simulink library "headingSetpointNumerical_cl"  (R2018b)
settings: Solver=VariableStepAuto  StartTime=0.0  StopTime=10.0  RelTol=1e-3
undefined symbols (not defined in the file): initialPathPosition_none
libraries: flatlandHeading_ul x1, offsetLeadDistance_ul x1, pathPositionNumerical_ul x1, pathProjectionNumerical_ul x1
settings Model: Creator=mcobb  LastModifiedBy=mitch
settings DebuggingCC: LibraryContextMissingDiagnostic=none
settings SFSimCC: SimUseLocalCustomCode=off
settings RTWCC: RTWUseLocalCustomCode=off

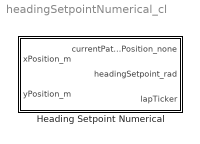
== system headingSetpointNumerical_cl ==
  Heading Setpoint Numerical : Subsystem

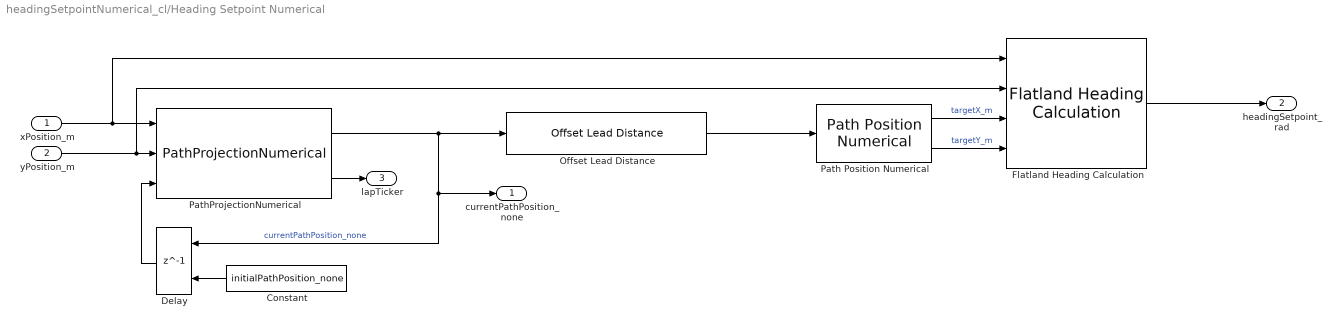
== system headingSetpointNumerical_cl/Heading Setpoint Numerical ==
  xPosition_m : Inport
  yPosition_m : Inport  Port=2
  Constant : Constant  Value=initialPathPosition_none
  Delay : Delay  DelayLength=1  InitialConditionSource=Input port  InitialCondition=0
      settings: InputPortMap=u0,p4
  Flatland Heading Calculation : flatlandHeading_ul/Flatland Heading Calculation  SystemSampleTime=-1
  Offset Lead Distance : offsetLeadDistance_ul/Offset Lead Distance  SystemSampleTime=-1
  Path Position Numerical : pathPositionNumerical_ul/Path Position Numerical  brkpts=projectionBreakpoints  xVals=projectionX  yVals=projectionY
  PathProjectionNumerical : pathProjectionNumerical_ul/PathProjectionNumerical  sDist=searchDistance_none  brkpts=projectionBreakpoints  xVals=projectionX  yVals=projectionY
  currentPathPosition_none : Outport
  headingSetpoint_rad : Outport  Port=2
  lapTicker : Outport  Port=3
  wires:
  Offset Lead Distance/1 -> Path Position Numerical/1
  Flatland Heading Calculation/1 -> headingSetpoint_rad/1
  PathProjectionNumerical/1 -> currentPathPosition_none/1, Delay/1, Offset Lead Distance/1  "currentPathPosition_none"
  Path Position Numerical/1 -> Flatland Heading Calculation/3  "targetX_m"
  Path Position Numerical/2 -> Flatland Heading Calculation/4  "targetY_m"
  xPosition_m/1 -> Flatland Heading Calculation/1, PathProjectionNumerical/1
  yPosition_m/1 -> Flatland Heading Calculation/2, PathProjectionNumerical/2
  Delay/1 -> PathProjectionNumerical/3
  Constant/1 -> Delay/2
  PathProjectionNumerical/2 -> lapTicker/1
